simulink subsystem "PieroG31Model"  (R2022b)
settings: Solver=VariableStepAuto  StartTime=0.0  StopTime=10.0  RelTol=1e-3
settings Model: Creator=dar.io  LastModifiedBy=dar.io

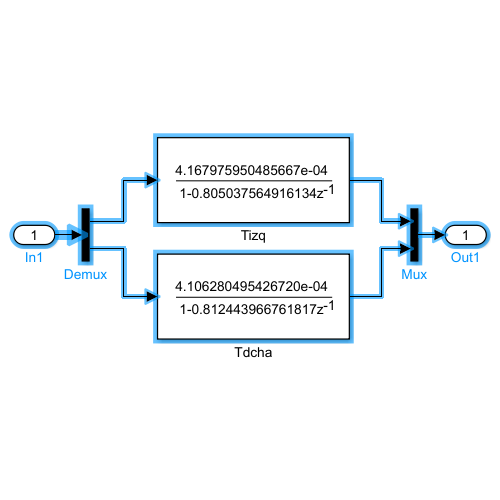
[thumbnail: Simulink's stored preview of the top-level diagram]
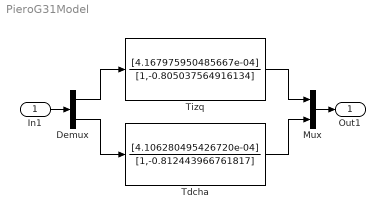
== system PieroG31Model ==
  In1 : Inport
  Demux : Demux  Outputs=2
  Mux : Mux  Inputs=2
  Tdcha : DiscreteFilter  Numerator=[4.106280495426720e-04]  Denominator=[1,-0.812443966761817]
  Tizq : DiscreteFilter  Numerator=[4.167975950485667e-04]  Denominator=[1,-0.805037564916134]
  Out1 : Outport
  wires:
  Tizq/1 -> Mux/1
  Demux/1 -> Tizq/1
  Tdcha/1 -> Mux/2
  Demux/2 -> Tdcha/1
  Mux/1 -> Out1/1
  In1/1 -> Demux/1
